simulink library "uavsimblockset"  (Simulink 8.6)
settings: Solver=ode45  StartTime=0.0  StopTime=10.0  RelTol=1e-3
undefined symbols (not defined in the file or in its folder): aircraftmask_displayVortices, aircraftmask_ID, DiscIntNeverNeededParam, uavsim
undefined symbols (not defined in the file): aircraftmask_originNED_ECEF_rrm, aircraftmask_p0_NED_m, aircraftmask_phithetapsi0, aircraftmask_pqr0, aircraftmask_uvw0, fflib_degdegm2rrm, flat2lla
libraries: uavsimBlockset_ServoHS55 x5, aerolibtransform2 x4, aerolibutil x3, uavsimBlockset_UAV3DInterface x3, uavsimblockset_SixDOFKinematics x2, simulink_extras x2, uavsimBlockset_Cularis_withUAV3D x2, uavsimBlockset_ElectricPropulsion x2, formationFlyingBlockset x2, uavsimBlockset_DerivedAerodynamicConditions x2, uavsimBlockset_alphabetaVa2uvw x1, uavsimBlockset_AirspeedController x1
(part 2 of 2)

== system uavsimblockset/Cularis aerodynamics/Aerodynamics/Aerodynamic Coefficients Cularis/Datum Coefficients/CL ==
  note: CL_0
  Alpha : Inport
  1 : Constant  Value=uavsim.CULARIS.CL_0
  CL_alpha : Gain  Gain=uavsim.CULARIS.CL_alpha
  Sum2 : Sum  Inputs=|++
  CL : Outport
  wires:
  1/1 -> Sum2/2
  Alpha/1 -> CL_alpha/1
  CL_alpha/1 -> Sum2/1
  Sum2/1 -> CL/1

== system uavsimblockset/Cularis aerodynamics/Aerodynamics/Aerodynamic Coefficients Cularis/Datum Coefficients/CY ==
  "Beta " : Inport
  "CY_0 " : Constant  Value=uavsim.CULARIS.CY_0
  CY_beta : Gain  Gain=uavsim.CULARIS.CY_beta  SaturateOnIntegerOverflow=on  OutDataTypeStr=Inherit: Same as input  ParamDataTypeStr=Inherit: Same as input
  Sum : Sum  Inputs=|++
  CY : Outport
  wires:
  "Beta "/1 -> CY_beta/1
  Sum/1 -> CY/1
  CY_beta/1 -> Sum/2
  "CY_0 "/1 -> Sum/1

== system uavsimblockset/Cularis aerodynamics/Aerodynamics/Aerodynamic Coefficients Cularis/Datum Coefficients/Cl ==
  Beta : Inport
  "Cl_0 " : Constant  Value=uavsim.CULARIS.Cl_0
  Cl_beta : Gain  Gain=uavsim.CULARIS.Cl_beta  SaturateOnIntegerOverflow=on  OutDataTypeStr=Inherit: Same as input  ParamDataTypeStr=Inherit: Same as input
  Sum1 : Sum  Inputs=|++
  "Cl " : Outport
  wires:
  Cl_beta/1 -> Sum1/1
  "Cl_0 "/1 -> Sum1/2
  Sum1/1 -> "Cl "/1
  Beta/1 -> Cl_beta/1

== system uavsimblockset/Cularis aerodynamics/Aerodynamics/Aerodynamic Coefficients Cularis/Datum Coefficients/Cm ==
  Alpha : Inport
  Cm_0 : Constant  Value=uavsim.CULARIS.Cm_0
  Cm_alpha : Gain  Gain=uavsim.CULARIS.Cm_alpha  SaturateOnIntegerOverflow=on  OutDataTypeStr=Inherit: Same as input  ParamDataTypeStr=Inherit: Same as input
  Sum2 : Sum  Inputs=|++
  Cm : Outport
  wires:
  Cm_0/1 -> Sum2/2
  Sum2/1 -> Cm/1
  Cm_alpha/1 -> Sum2/1
  Alpha/1 -> Cm_alpha/1

== system uavsimblockset/Cularis aerodynamics/Aerodynamics/Aerodynamic Coefficients Cularis/Datum Coefficients/Cn ==
  Beta : Inport
  Cn_0 : Constant  Value=uavsim.CULARIS.Cn_0
  Cn_beta : Gain  Gain=uavsim.CULARIS.Cn_beta  SaturateOnIntegerOverflow=on  OutDataTypeStr=Inherit: Same as input  ParamDataTypeStr=Inherit: Same as input
  Sum3 : Sum  Inputs=|++
  Cn : Outport
  wires:
  Cn_0/1 -> Sum3/2
  Sum3/1 -> Cn/1
  Cn_beta/1 -> Sum3/1
  Beta/1 -> Cn_beta/1

== matlab function Publish state/MATLAB Function1 ==
  data: pNED input double; vNED input double; CL input double; qAttitude input double; alpha input double; beta input double; p input double; tsim input double; VortexSig data_store_memory double
% This function writes the calling aircraft's relevant states into a global
% Simulink variable to enable Simulation of relative localization sensors,
% aerodynamic coupling etc.
function publishState(pNED, ...
    vNED, ...
    CL, ...
    qAttitude, ...
    alpha, ...
    beta, ...
    p, ...
    tsim)
%#codegen
global VortexSig;

ID = p.id;
VortexSig(ID).timeOfLastUpdate = tsim;
VortexSig(ID).p_NED_m = pNED;
VortexSig(ID).v_NED_mps = vNED;
VortexSig(ID).CL = CL;
VortexSig(ID).qAttitude = qAttitude;
VortexSig(ID).alpha_rad = alpha;
VortexSig(ID).beta_rad = beta;
VortexSig(ID).b_m = p.b_m;

VortexSig(ID).cbar_m = p.cbar_m;
VortexSig(ID).sweep_rad = p.sweep_rad;
VortexSig(ID).dihedral_rad = p.dihedral_rad;
VortexSig(ID).longiRefLength_m = p.longiRefLength_m;
VortexSig(ID).pNose_b_m = p.pNose_b_m;
VortexSig(ID).pRear_b_m = [-1/4 0 0]';
VortexSig(ID).posFuselageBottom_b_m = [0 0 0.12/2]';
VortexSig(ID).verticalRefLength_m = p.verticalRefLength_m;
VortexSig(ID).posFinTip_b_m = p.posFinTip_b_m;

end

== matlab function Closed loop Cularis UAS 1/Controllers/Subsystem/Compute differential positions and velocities ==
  data: dx output Bus: Dx; closedloopmask_ID parameter double; VortexSig data_store_memory double
function dx = fcn(closedloopmask_ID)
%#codegen
global VortexSig;

dx = struct('dp_NED_m', zeros(10,3), 'dv_NED_mps', zeros(10,3));

for k=1:10
   dx.dp_NED_m(k, :) = VortexSig(k).p_NED_m - VortexSig(closedloopmask_ID).p_NED_m;
   dx.dv_NED_mps(k, :) = VortexSig(k).v_NED_mps - VortexSig(closedloopmask_ID).v_NED_mps;
end

end

== matlab function Closed loop Cularis UAS 1/Controllers/Compute error measures/Compute differential positions and velocities ==
  data: dx output Bus: Dx; closedloopmask_ID parameter double; VortexSig data_store_memory double; dt output double
function [dx, dt] = fcn(closedloopmask_ID)
%#codegen
global VortexSig;

dx = struct('dp_NED_m', zeros(10,3), 'dv_NED_mps', zeros(10,3));
dt = zeros(10,1);
for k=1:10
   dx.dp_NED_m(k, :) = VortexSig(k).p_NED_m - VortexSig(closedloopmask_ID).p_NED_m;
   dx.dv_NED_mps(k, :) = VortexSig(k).v_NED_mps - VortexSig(closedloopmask_ID).v_NED_mps;
   dt(k, :) = VortexSig(k).timeOfLastUpdate - VortexSig(closedloopmask_ID).timeOfLastUpdate;   
end

end
